simulink model "TRR_LQR"  (R2020a)
settings: Solver=VariableStepAuto  StartTime=0.0  StopTime=10  RelTol=1e-3
values from neighbouring files (symbols this model uses):
  A = [0 0 0 1 0 0 ... (first row only)    [TRR_PID_parameters.m]
  B = [0 0 0 ... (first row only)    [TRR_PID_parameters.m]
  G = [g*m3*cos(theta1)*(a3*cos(theta2 + theta3) + a2*cos(theta2)) + a2*g*m2*cos(theta1)*cos(theta2) ... (first row only)    [TRR_PID_parameters.m]
  JT = transpose(J)    [TRR_PID_parameters.m]
  M = [((m3*(a2^2*cos(2*theta2)+a3^2*cos(2*theta2+2*theta3)+a2^2+a3^2+2*a2*a3*cos(2*theta2+theta3)+2*a2*a3*cos(theta3)))/2+m2*a2*a2*cos(theta2)^2) 0 0 ... (first row only)    [TRR_PID_parameters.m]
  theta1 = atand(y/x) - phi1    [IK_RR.m]    (also in IK_TRR.m = atan(y/x); TRR_PID_parameters.m = atan(y/x))
  theta2 = 180 - phi2    [IK_RR.m]    (also in IK_TRR.m = 1.57079632679; TRR_PID_parameters.m = -1.57079632679)
  theta21 = real(Theta21), theta22 = real(Theta22), theta23 = real(Theta23)    [TRR_PID_parameters.m]
  theta3 = -(pi - phi3)    [IK_TRR.m]    (also in TRR_PID_parameters.m = pi - phi3)
  V1 = [0 0.5*(-theta1_dot*(a3^2*m3*sin(2*theta2 + 2*theta3)+a2^2*m3*sin(2*theta2)+2*a2*a3*m3*sin(2*theta2 + theta3)+2*a2^2*m2*cos(theta2)*sin(theta2))) 0.5*(-theta1_dot*(a3^2*m3*sin(2*theta2 + 2*theta3) + a2*a3*m3*sin(2*theta2 + theta3) + a2*a3*m3*sin(theta3))) ... (first row only)    [TRR_PID_parameters.m]
undefined symbols (not defined in the file or in its folder): B_imp, K, K_imp, tau1, tau2, tau3, theta22, theta23
libraries: simulink x4
settings Model: Creator=Dr.Saraf  LastModifiedBy=Dr.Saraf

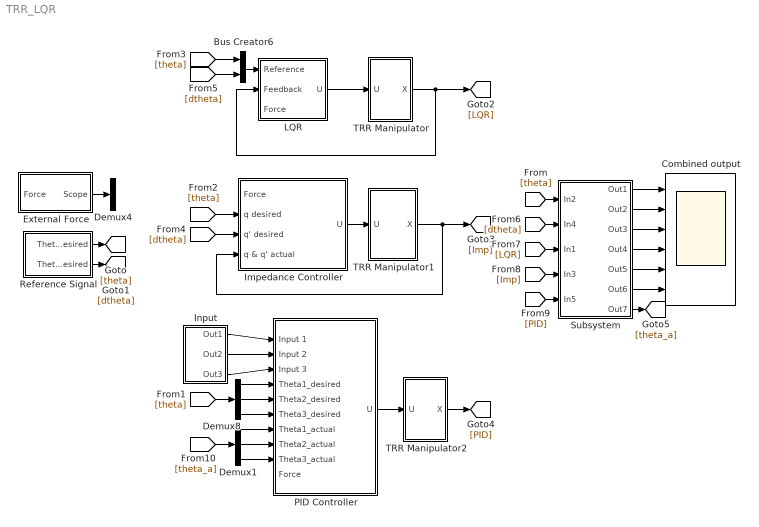
== system TRR_LQR ==
  Bus Creator6 : BusCreator  Inputs=2
  Combined output : Scope  NumInputPorts=6
  Demux1 : Demux  Outputs=3
  Demux4 : Demux  Outputs=3
  Demux8 : Demux  Outputs=3
  External Force : Subsystem
      settings: PortSchema="{\"entries\":[{\"content\":{\"sides\":[{\"content\":{\"connectorIds\":[\"Out2\"]},\"type\":\"ConnectorPlacement.EquallySpacedRectSide\",\"uuid\":\"bc6f37bf-b6c5-4028-b4a4-1f6ac3343290\"},{\"content\":{\"connectorIds\":[\"Out1\"],\"side\":\"RIGHT\"},\"type\":\"ConnectorPlacement.EquallySpacedRectSide\",\"uuid\":\"4c1d6f8d-9a15-4436-8744-0df7d527871c\"},{\"content\":{\"connectorIds\":[],\"side\":\"TOP\"},\"type\":\"ConnectorPlacement.EquallySpacedRectSide\",\"uuid\":\"b806ddfa-c017-4b4f-bf2f-a13602b353a7\"}]},\"type\":\"ConnectorPlacement.EquallySpacedConnector\",\"uuid\":\"efa4b6a4-9e82-4f59-9dc9-02b8956516e8\"}],\"packageUris\":[\"http://schema.mathworks.com/mf0/Connector/19700101\"],\"version\":\"1.0\"}"
  Impedance Controller : Subsystem
  Input : Subsystem
  LQR : Subsystem
  PID Controller : Subsystem
  Reference Signal : Subsystem
  Subsystem : Subsystem
  TRR Manipulator : Subsystem
  TRR Manipulator1 : Subsystem
      mask Display: image('Manipulator.jpg'); % Use "Edit Image" on toolstrip to change.
  TRR Manipulator2 : Subsystem
  wires:
  LQR/1(U) -> TRR Manipulator/1(U)
  External Force/1(Scope) -> Demux4/1
  Impedance Controller/1(U) -> TRR Manipulator1/1(U)
  Bus Creator6/1 -> LQR/1(Reference)
  Input/3(Out3) -> PID Controller/3(Input 3)
  Input/2(Out2) -> PID Controller/2(Input 2)
  Input/1(Out1) -> PID Controller/1(Input 1)
  Demux8/1 -> PID Controller/4(Theta1_desired)
  Demux8/2 -> PID Controller/5(Theta2_desired)
  Demux8/3 -> PID Controller/6(Theta3_desired)
  TRR Manipulator1/1(X) -> Impedance Controller/4(q & q' actual), [Imp]
  TRR Manipulator/1(X) -> [LQR], LQR/2(Feedback)
  Subsystem/1(Out1) -> Combined output/1
  Subsystem/2(Out2) -> Combined output/2
  Subsystem/3(Out3) -> Combined output/3
  Subsystem/4(Out4) -> Combined output/4
  Subsystem/5(Out5) -> Combined output/5
  Subsystem/6(Out6) -> Combined output/6
  Demux1/1 -> PID Controller/7(Theta1_actual)
  Demux1/2 -> PID Controller/8(Theta2_actual)
  Demux1/3 -> PID Controller/9(Theta3_actual)
  Reference Signal/1(Theta_desired) -> [theta]
  [theta] -> Bus Creator6/1
  [theta] -> Impedance Controller/2(q desired)
  [theta] -> Demux8/1
  [theta] -> Subsystem/1(In2)
  Reference Signal/2(Theta'_desired) -> [dtheta]
  [dtheta] -> Subsystem/2(In4)
  [dtheta] -> Bus Creator6/2
  [dtheta] -> Impedance Controller/3(q' desired)
  [LQR] -> Subsystem/3(In1)
  [Imp] -> Subsystem/4(In3)
  [PID] -> Subsystem/5(In5)
  TRR Manipulator2/1(X) -> [PID]
  PID Controller/1(U) -> TRR Manipulator2/1(U)
  [theta_a] -> Demux1/1
  Subsystem/7(Out7) -> [theta_a]

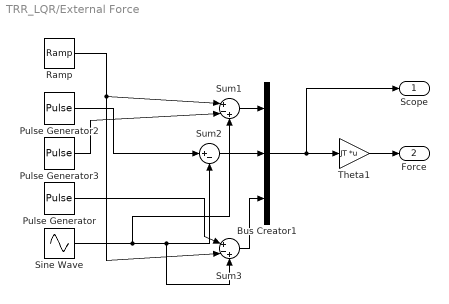
== system TRR_LQR/External Force ==
  Bus Creator1 : BusCreator  Inputs=3
  Pulse Generator : DiscretePulseGenerator  PulseType=Time based  Amplitude=15  Period=5  PulseWidth=5
  Pulse Generator2 : DiscretePulseGenerator  PulseType=Time based  Amplitude=10  Period=10  PulseWidth=20
  Pulse Generator3 : DiscretePulseGenerator  PulseType=Time based  Amplitude=20  Period=10  PulseWidth=10  PhaseDelay=4
  Ramp : simulink/Sources/Ramp  slope=2  start=0  InitialOutput=0
  Sine Wave : Sin  Amplitude=2  Frequency=2  SampleTime=0
  Sum1 : Sum  Inputs=|+-+
  Sum2 : Sum  Inputs=|+-
  Sum3 : Sum  Inputs=|+-+
  Theta1 : Gain  Gain=JT  Multiplication=Matrix(K*u)
  Scope : Outport
  Force : Outport  Port=2
  wires:
  Bus Creator1/1 -> Scope/1, Theta1/1
  Theta1/1 -> Force/1
  Pulse Generator/1 -> Sum3/1
  Pulse Generator3/1 -> Sum1/2
  Ramp/1 -> Sum3/2, Sum1/1
  Pulse Generator2/1 -> Sum2/1
  Sine Wave/1 -> Sum1/3, Sum3/3, Sum2/2
  Sum3/1 -> Bus Creator1/3
  Sum2/1 -> Bus Creator1/2
  Sum1/1 -> Bus Creator1/1

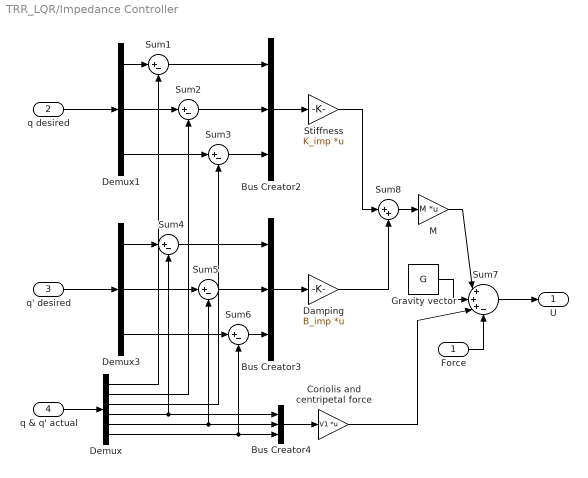
== system TRR_LQR/Impedance Controller ==
  Force : Inport
  q desired : Inport  Port=2
  q' desired : Inport  Port=3
  q & q' actual : Inport  Port=4
  Bus Creator2 : BusCreator  Inputs=3
  Bus Creator3 : BusCreator  Inputs=3
  Bus Creator4 : BusCreator  Inputs=3
  Coriolis and centripetal force : Gain  Gain=V1  Multiplication=Matrix(K*u)
  Damping : Gain  Gain=B_imp  Multiplication=Matrix(K*u)
  Demux : Demux  Outputs=6
  Demux1 : Demux  Outputs=3
  Demux3 : Demux  Outputs=3
  Gravity vector : Constant  Value=G  VectorParams1D=off
  M : Gain  Gain=M  Multiplication=Matrix(K*u)
  Stiffness : Gain  Gain=K_imp  Multiplication=Matrix(K*u)
  Sum{1..6} (6 alike) : Sum  Inputs=|+-
  Sum7 : Sum  Inputs=|+++-
  Sum8 : Sum  Inputs=|++
  U : Outport
  wires:
  Sum8/1 -> M/1
  Sum6/1 -> Bus Creator3/3
  Stiffness/1 -> Sum8/1
  Demux/3 -> Sum3/2
  Sum1/1 -> Bus Creator2/1
  Force/1 -> Sum7/4
  Bus Creator4/1 -> Coriolis and centripetal force/1
  Bus Creator2/1 -> Stiffness/1
  Demux/5 -> Bus Creator4/2, Sum5/2
  Sum5/1 -> Bus Creator3/2
  Demux/4 -> Bus Creator4/1, Sum4/2
  Demux/6 -> Bus Creator4/3, Sum6/2
  Sum2/1 -> Bus Creator2/2
  Demux/1 -> Sum1/2
  Bus Creator3/1 -> Damping/1
  Sum4/1 -> Bus Creator3/1
  Demux3/1 -> Sum4/1
  Sum3/1 -> Bus Creator2/3
  Demux/2 -> Sum2/2
  M/1 -> Sum7/1
  Damping/1 -> Sum8/2
  Demux3/3 -> Sum6/1
  q & q' actual/1 -> Demux/1
  Sum7/1 -> U/1
  Demux1/3 -> Sum3/1
  Demux1/1 -> Sum1/1
  Demux1/2 -> Sum2/1
  Demux3/2 -> Sum5/1
  Gravity vector/1 -> Sum7/2
  Coriolis and centripetal force/1 -> Sum7/3
  q desired/1 -> Demux1/1
  q' desired/1 -> Demux3/1

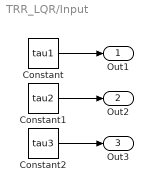
== system TRR_LQR/Input ==
  Constant : Constant  Value=tau1
  Constant1 : Constant  Value=tau2
  Constant2 : Constant  Value=tau3
  Out1 : Outport
  Out2 : Outport  Port=2
  Out3 : Outport  Port=3
  wires:
  Constant1/1 -> Out2/1
  Constant2/1 -> Out3/1
  Constant/1 -> Out1/1

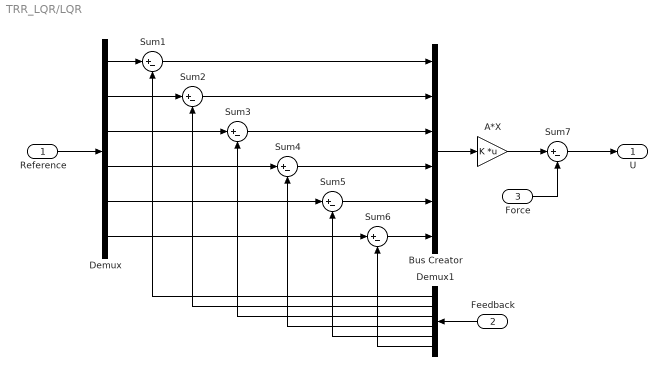
== system TRR_LQR/LQR ==
  Reference : Inport
  Feedback : Inport  Port=2
  Force : Inport  Port=3
  A*X : Gain  Gain=K  Multiplication=Matrix(K*u)
  Bus Creator : BusCreator  Inputs=6
  Demux : Demux  Outputs=6
  Demux1 : Demux  Outputs=6
  Sum{1..7} (7 alike) : Sum  Inputs=|+-
  U : Outport
  wires:
  Bus Creator/1 -> A*X/1
  Sum2/1 -> Bus Creator/2
  Sum6/1 -> Bus Creator/6
  Sum3/1 -> Bus Creator/3
  Sum5/1 -> Bus Creator/5
  Sum4/1 -> Bus Creator/4
  Demux/6 -> Sum6/1
  Demux1/5 -> Sum5/2
  Demux1/3 -> Sum3/2
  Demux1/2 -> Sum2/2
  Demux/1 -> Sum1/1
  Sum1/1 -> Bus Creator/1
  Demux1/4 -> Sum4/2
  Demux1/6 -> Sum6/2
  Demux/2 -> Sum2/1
  Demux1/1 -> Sum1/2
  Feedback/1 -> Demux1/1
  Demux/3 -> Sum3/1
  Demux/5 -> Sum5/1
  Demux/4 -> Sum4/1
  Reference/1 -> Demux/1
  A*X/1 -> Sum7/1
  Sum7/1 -> U/1
  Force/1 -> Sum7/2

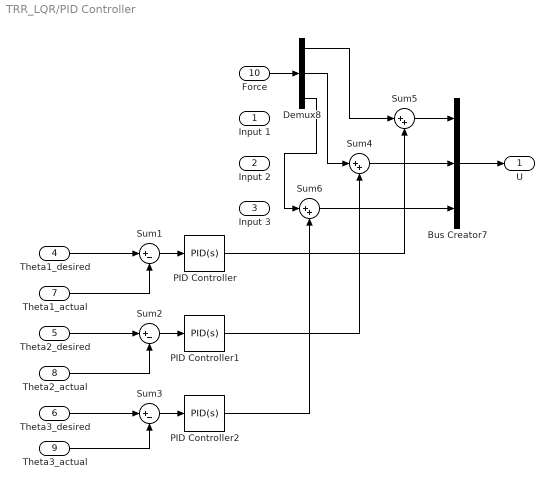
== system TRR_LQR/PID Controller ==
  Input 1 : Inport
  Input 2 : Inport  Port=2
  Input 3 : Inport  Port=3
  Theta1_desired : Inport  Port=4
  Theta2_desired : Inport  Port=5
  Theta3_desired : Inport  Port=6
  Theta1_actual : Inport  Port=7
  Theta2_actual : Inport  Port=8
  Theta3_actual : Inport  Port=9
  Force : Inport  Port=10
  Bus Creator7 : BusCreator  Inputs=3
  Demux8 : Demux  Outputs=3
  PID Controller : simulink/Continuous/PID Controller  Controller=PID  Form=Parallel  TimeDomain=Continuous-time  UseExternalTs=off  SampleTime=-1  IntegratorMethod=Forward Euler  FilterMethod=Forward Euler  ControllerParametersSource=internal  P=9385.78381494032  I=4216.64131274758  D=5201.3331364466  UseFilter=on  N=1142.8279760416  TunerSelectOption=Transfer Function Based (PID Tuner App)  InitialConditionSource=internal  InitialConditionForIntegrator=0  InitialConditionForFilter=0  DifferentiatorICPrevScaledInput=0  ExternalReset=none  TrackingMode=off  Kt=1  LimitOutput=off  UpperSaturationLimit=inf  LowerSaturationLimit=-inf  LinearizeAsGain=on  AntiWindupMode=none  Kb=1  POutMin=[]  POutMax=[]  IOutMin=[]  IOutMax=[]  DOutMin=[]  DOutMax=[]  NOutMin=[]  NOutMax=[]  SumOutMin=[]  SumOutMax=[]  SaturationOutMin=[]  SaturationOutMax=[]  PParamMin=[]  PParamMax=[]  IParamMin=[]  IParamMax=[]  DParamMin=[]  DParamMax=[]  NParamMin=[]  NParamMax=[]  KbParamMin=[]  KbParamMax=[]  KtParamMin=[]  KtParamMax=[]  KbOutMin=[]  KbOutMax=[]  KtOutMin=[]  KtOutMax=[]  IntegratorOutMin=[]  IntegratorOutMax=[]  FilterOutMin=[]  FilterOutMax=[]  SumI1OutMin=[]  SumI1OutMax=[]  SumI2OutMin=[]  SumI2OutMax=[]  SumI3OutMin=[]  SumI3OutMax=[]  SumI4OutMin=[]  SumI4OutMax=[]  SumDOutMin=[]  SumDOutMax=[]  DifferentiatorOutMin=[]  DifferentiatorOutMax=[]  FilterDiffOutCoefMin=[]  FilterDiffOutCoefMax=[]  ReciprocalOutMin=[]  ReciprocalOutMax=[]  SumDenOutMin=[]  SumDenOutMax=[]  SumNumOutMin=[]  SumNumOutMax=[]  DivideOutMin=[]  DivideOutMax=[]  UdiffTsProdOutMin=[]  UdiffTsProdOutMax=[]  NTsProdOutMin=[]  NTsProdOutMax=[]  UintegralTsProdOutMin=[]  UintegralTsProdOutMax=[]  UngainTsProdOutMin=[]  UngainTsProdOutMax=[]  IntegratorContinuousStateAttributes=''  IntegratorStateMustResolveToSignalObject=off  IntegratorRTWStateStorageClass=Auto  FilterContinuousStateAttributes=''  FilterStateMustResolveToSignalObject=off  FilterRTWStateStorageClass=Auto  ParallelPVariant=InternalParameters  IdealPVariant=Disabled  IVariant=InternalParameters  DVariant=InternalParameters  IntegratorVariant=Continuous  SatVariant=Disabled  AWVariant=Passthrough  PCopyVariant=Disabled  TRVariant=Disabled  FdbkBlocksVariant=Forward  IdealPFdbkVariant=Disabled  SatFdbkVariant=Disabled  DerivativeFilterVariant=ContFilter  NVariant=InternalParameters  NCopyVariant=Disabled  FilterICVariant=InternalICsFilter  IntegratorICVariant=InternalICs  ExternalResetVariant=Disabled  TRSumVariant=Passthrough  SumFdbkVariant=Disabled  SumVariant=Sum_PID  TsampFilterVariant=InternalTs  TsampNgainVariant=Passthrough  TsampIntegralVariant=Passthrough
  PID Controller1 : simulink/Continuous/PID Controller  Controller=PID  Form=Parallel  TimeDomain=Continuous-time  UseExternalTs=off  SampleTime=-1  IntegratorMethod=Forward Euler  FilterMethod=Forward Euler  ControllerParametersSource=internal  P=492.875843269351  I=550.092822948062  D=75.3098650397504  UseFilter=on  N=6127.40225681107  TunerSelectOption=Transfer Function Based (PID Tuner App)  InitialConditionSource=internal  InitialConditionForIntegrator=0  InitialConditionForFilter=0  DifferentiatorICPrevScaledInput=0  ExternalReset=none  TrackingMode=off  Kt=1  LimitOutput=off  UpperSaturationLimit=inf  LowerSaturationLimit=-inf  LinearizeAsGain=on  AntiWindupMode=none  Kb=1  POutMin=[]  POutMax=[]  IOutMin=[]  IOutMax=[]  DOutMin=[]  DOutMax=[]  NOutMin=[]  NOutMax=[]  SumOutMin=[]  SumOutMax=[]  SaturationOutMin=[]  SaturationOutMax=[]  PParamMin=[]  PParamMax=[]  IParamMin=[]  IParamMax=[]  DParamMin=[]  DParamMax=[]  NParamMin=[]  NParamMax=[]  KbParamMin=[]  KbParamMax=[]  KtParamMin=[]  KtParamMax=[]  KbOutMin=[]  KbOutMax=[]  KtOutMin=[]  KtOutMax=[]  IntegratorOutMin=[]  IntegratorOutMax=[]  FilterOutMin=[]  FilterOutMax=[]  SumI1OutMin=[]  SumI1OutMax=[]  SumI2OutMin=[]  SumI2OutMax=[]  SumI3OutMin=[]  SumI3OutMax=[]  SumI4OutMin=[]  SumI4OutMax=[]  SumDOutMin=[]  SumDOutMax=[]  DifferentiatorOutMin=[]  DifferentiatorOutMax=[]  FilterDiffOutCoefMin=[]  FilterDiffOutCoefMax=[]  ReciprocalOutMin=[]  ReciprocalOutMax=[]  SumDenOutMin=[]  SumDenOutMax=[]  SumNumOutMin=[]  SumNumOutMax=[]  DivideOutMin=[]  DivideOutMax=[]  UdiffTsProdOutMin=[]  UdiffTsProdOutMax=[]  NTsProdOutMin=[]  NTsProdOutMax=[]  UintegralTsProdOutMin=[]  UintegralTsProdOutMax=[]  UngainTsProdOutMin=[]  UngainTsProdOutMax=[]  IntegratorContinuousStateAttributes=''  IntegratorStateMustResolveToSignalObject=off  IntegratorRTWStateStorageClass=Auto  FilterContinuousStateAttributes=''  FilterStateMustResolveToSignalObject=off  FilterRTWStateStorageClass=Auto  ParallelPVariant=InternalParameters  IdealPVariant=Disabled  IVariant=InternalParameters  DVariant=InternalParameters  IntegratorVariant=Continuous  SatVariant=Disabled  AWVariant=Passthrough  PCopyVariant=Disabled  TRVariant=Disabled  FdbkBlocksVariant=Forward  IdealPFdbkVariant=Disabled  SatFdbkVariant=Disabled  DerivativeFilterVariant=ContFilter  NVariant=InternalParameters  NCopyVariant=Disabled  FilterICVariant=InternalICsFilter  IntegratorICVariant=InternalICs  ExternalResetVariant=Disabled  TRSumVariant=Passthrough  SumFdbkVariant=Disabled  SumVariant=Sum_PID  TsampFilterVariant=InternalTs  TsampNgainVariant=Passthrough  TsampIntegralVariant=Passthrough
  PID Controller2 : simulink/Continuous/PID Controller  Controller=PID  Form=Parallel  TimeDomain=Continuous-time  UseExternalTs=off  SampleTime=-1  IntegratorMethod=Forward Euler  FilterMethod=Forward Euler  ControllerParametersSource=internal  P=776.91774371063  I=154.631169300586  D=867.309317025399  UseFilter=on  N=3898.89672467147  TunerSelectOption=Transfer Function Based (PID Tuner App)  InitialConditionSource=internal  InitialConditionForIntegrator=0  InitialConditionForFilter=0  DifferentiatorICPrevScaledInput=0  ExternalReset=none  TrackingMode=off  Kt=1  LimitOutput=off  UpperSaturationLimit=inf  LowerSaturationLimit=-inf  LinearizeAsGain=on  AntiWindupMode=none  Kb=1  POutMin=[]  POutMax=[]  IOutMin=[]  IOutMax=[]  DOutMin=[]  DOutMax=[]  NOutMin=[]  NOutMax=[]  SumOutMin=[]  SumOutMax=[]  SaturationOutMin=[]  SaturationOutMax=[]  PParamMin=[]  PParamMax=[]  IParamMin=[]  IParamMax=[]  DParamMin=[]  DParamMax=[]  NParamMin=[]  NParamMax=[]  KbParamMin=[]  KbParamMax=[]  KtParamMin=[]  KtParamMax=[]  KbOutMin=[]  KbOutMax=[]  KtOutMin=[]  KtOutMax=[]  IntegratorOutMin=[]  IntegratorOutMax=[]  FilterOutMin=[]  FilterOutMax=[]  SumI1OutMin=[]  SumI1OutMax=[]  SumI2OutMin=[]  SumI2OutMax=[]  SumI3OutMin=[]  SumI3OutMax=[]  SumI4OutMin=[]  SumI4OutMax=[]  SumDOutMin=[]  SumDOutMax=[]  DifferentiatorOutMin=[]  DifferentiatorOutMax=[]  FilterDiffOutCoefMin=[]  FilterDiffOutCoefMax=[]  ReciprocalOutMin=[]  ReciprocalOutMax=[]  SumDenOutMin=[]  SumDenOutMax=[]  SumNumOutMin=[]  SumNumOutMax=[]  DivideOutMin=[]  DivideOutMax=[]  UdiffTsProdOutMin=[]  UdiffTsProdOutMax=[]  NTsProdOutMin=[]  NTsProdOutMax=[]  UintegralTsProdOutMin=[]  UintegralTsProdOutMax=[]  UngainTsProdOutMin=[]  UngainTsProdOutMax=[]  IntegratorContinuousStateAttributes=''  IntegratorStateMustResolveToSignalObject=off  IntegratorRTWStateStorageClass=Auto  FilterContinuousStateAttributes=''  FilterStateMustResolveToSignalObject=off  FilterRTWStateStorageClass=Auto  ParallelPVariant=InternalParameters  IdealPVariant=Disabled  IVariant=InternalParameters  DVariant=InternalParameters  IntegratorVariant=Continuous  SatVariant=Disabled  AWVariant=Passthrough  PCopyVariant=Disabled  TRVariant=Disabled  FdbkBlocksVariant=Forward  IdealPFdbkVariant=Disabled  SatFdbkVariant=Disabled  DerivativeFilterVariant=ContFilter  NVariant=InternalParameters  NCopyVariant=Disabled  FilterICVariant=InternalICsFilter  IntegratorICVariant=InternalICs  ExternalResetVariant=Disabled  TRSumVariant=Passthrough  SumFdbkVariant=Disabled  SumVariant=Sum_PID  TsampFilterVariant=InternalTs  TsampNgainVariant=Passthrough  TsampIntegralVariant=Passthrough
  Sum1 : Sum  Inputs=|+-
  Sum2 : Sum  Inputs=|+-
  Sum3 : Sum  Inputs=|+-
  Sum4 : Sum  Inputs=|++
  Sum5 : Sum  Inputs=|++
  Sum6 : Sum  Inputs=|++
  U : Outport
  wires:
  Sum1/1 -> PID Controller/1
  Sum2/1 -> PID Controller1/1
  Sum3/1 -> PID Controller2/1
  Theta3_actual/1 -> Sum3/2
  Theta1_actual/1 -> Sum1/2
  Theta3_desired/1 -> Sum3/1
  Theta2_desired/1 -> Sum2/1
  Theta2_actual/1 -> Sum2/2
  Theta1_desired/1 -> Sum1/1
  PID Controller/1 -> Sum5/2
  PID Controller1/1 -> Sum4/2
  PID Controller2/1 -> Sum6/2
  Force/1 -> Demux8/1
  Demux8/1 -> Sum5/1
  Demux8/2 -> Sum4/1
  Demux8/3 -> Sum6/1
  Bus Creator7/1 -> U/1
  Sum5/1 -> Bus Creator7/1
  Sum4/1 -> Bus Creator7/2
  Sum6/1 -> Bus Creator7/3

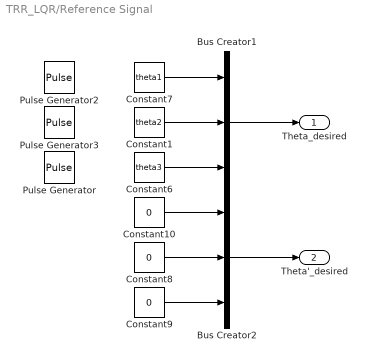
== system TRR_LQR/Reference Signal ==
  Bus Creator1 : BusCreator  Inputs=3
  Bus Creator2 : BusCreator  Inputs=3
  Constant1 : Constant  Value=theta2
  Constant10 : Constant  Value=0
  Constant6 : Constant  Value=theta3
  Constant7 : Constant  Value=theta1
  Constant8 : Constant  Value=0
  Constant9 : Constant  Value=0
  Pulse Generator : DiscretePulseGenerator  PulseType=Time based  Amplitude=theta23  Period=5  PulseWidth=50
  Pulse Generator2 : DiscretePulseGenerator  PulseType=Time based  Amplitude=theta21  Period=5  PulseWidth=50
  Pulse Generator3 : DiscretePulseGenerator  PulseType=Time based  Amplitude=theta22  Period=5  PulseWidth=50
  Theta_desired : Outport
  Theta'_desired : Outport  Port=2
  wires:
  Constant9/1 -> Bus Creator2/3
  Constant8/1 -> Bus Creator2/2
  Constant10/1 -> Bus Creator2/1
  Bus Creator1/1 -> Theta_desired/1
  Bus Creator2/1 -> Theta'_desired/1
  Constant7/1 -> Bus Creator1/1
  Constant1/1 -> Bus Creator1/2
  Constant6/1 -> Bus Creator1/3

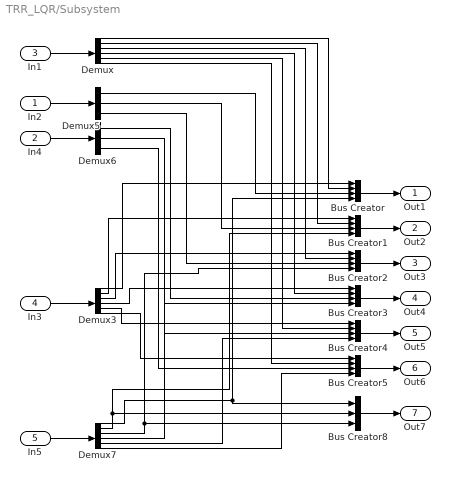
== system TRR_LQR/Subsystem ==
  In2 : Inport
  In4 : Inport  Port=2
  In1 : Inport  Port=3
  In3 : Inport  Port=4
  In5 : Inport  Port=5
  Bus Creator{,1..5} (6 alike) : BusCreator  Inputs=4
  Bus Creator8 : BusCreator  Inputs=3
  Demux : Demux  Outputs=6
  Demux3 : Demux  Outputs=6
  Demux5 : Demux  Outputs=3
  Demux6 : Demux  Outputs=3
  Demux7 : Demux  Outputs=6
  Out1 : Outport
  Out2 : Outport  Port=2
  Out3 : Outport  Port=3
  Out4 : Outport  Port=4
  Out5 : Outport  Port=5
  Out6 : Outport  Port=6
  Out7 : Outport  Port=7
  wires:
  Demux3/1 -> Bus Creator/1
  Demux3/2 -> Bus Creator1/1
  In2/1 -> Demux5/1
  Demux7/3 -> Bus Creator2/4, Bus Creator8/3
  In3/1 -> Demux3/1
  Demux7/2 -> Bus Creator8/2, Bus Creator1/4
  Demux/3 -> Bus Creator2/2
  Demux5/1 -> Bus Creator/3
  Demux/2 -> Bus Creator1/2
  In5/1 -> Demux7/1
  Bus Creator1/1 -> Out2/1
  Demux/1 -> Bus Creator/2
  Demux/5 -> Bus Creator4/2
  Demux6/1 -> Bus Creator3/3
  Demux3/5 -> Bus Creator4/1
  Demux3/6 -> Bus Creator5/1
  Demux3/4 -> Bus Creator3/1
  Demux/4 -> Bus Creator3/2
  Demux/6 -> Bus Creator5/2
  Demux7/4 -> Bus Creator3/4
  Demux3/3 -> Bus Creator2/1
  Demux7/1 -> Bus Creator8/1, Bus Creator/4
  Bus Creator4/1 -> Out5/1
  Bus Creator2/1 -> Out3/1
  Demux5/3 -> Bus Creator2/3
  Demux6/2 -> Bus Creator4/3
  Demux6/3 -> Bus Creator5/3
  Demux5/2 -> Bus Creator1/3
  Demux7/6 -> Bus Creator5/4
  Demux7/5 -> Bus Creator4/4
  In1/1 -> Demux/1
  Bus Creator8/1 -> Out7/1
  In4/1 -> Demux6/1
  Bus Creator5/1 -> Out6/1
  Bus Creator3/1 -> Out4/1
  Bus Creator/1 -> Out1/1

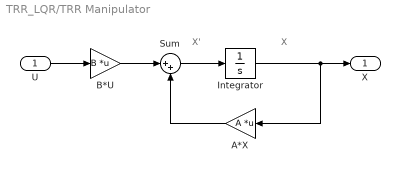
== system TRR_LQR/TRR Manipulator ==
  note: X'
  note: X
  U : Inport
  A*X : Gain  Gain=A  Multiplication=Matrix(K*u)
  B*U : Gain  Gain=B  Multiplication=Matrix(K*u)
  Integrator : Integrator  InitialCondition=[0, 0, 0, 0, 0, 0]
  Sum : Sum  Inputs=|++
  X : Outport
  wires:
  Integrator/1 -> X/1, A*X/1
  B*U/1 -> Sum/1
  Sum/1 -> Integrator/1
  A*X/1 -> Sum/2
  U/1 -> B*U/1

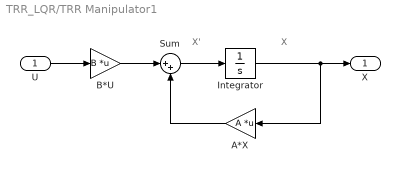
== system TRR_LQR/TRR Manipulator1 ==
  note: X'
  note: X
  U : Inport
  A*X : Gain  Gain=A  Multiplication=Matrix(K*u)
  B*U : Gain  Gain=B  Multiplication=Matrix(K*u)
  Integrator : Integrator  InitialCondition=[0; 0; 0; 0; 0; 0]
  Sum : Sum  Inputs=|++
  X : Outport
  wires:
  Integrator/1 -> X/1, A*X/1
  B*U/1 -> Sum/1
  Sum/1 -> Integrator/1
  A*X/1 -> Sum/2
  U/1 -> B*U/1

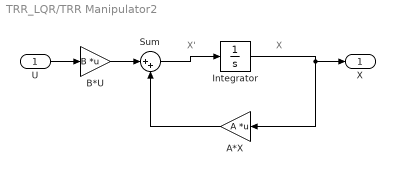
== system TRR_LQR/TRR Manipulator2 ==
  note: X'
  note: X
  U : Inport
  A*X : Gain  Gain=A  Multiplication=Matrix(K*u)
  B*U : Gain  Gain=B  Multiplication=Matrix(K*u)
  Integrator : Integrator  InitialCondition=[0, 0, 0, 0, 0, 0]
  Sum : Sum  Inputs=|++
  X : Outport
  wires:
  Integrator/1 -> A*X/1, X/1
  B*U/1 -> Sum/1
  Sum/1 -> Integrator/1
  A*X/1 -> Sum/2
  U/1 -> B*U/1
